simulink model "LQI_tests"  (R2026a)
settings: Solver=FixedStepAuto  StopTime=60  FixedStep=1e-3  RelTol=1e-5
values from neighbouring files (symbols this model uses):
  g = p.g    [HopperLinearization_6DOF.m]    (also in HopperLinearization_6DOF_LQR.m; HopperLinearization_6DOF_inertial.m; HopperLinearization_errorq.m; TetherTrajectory.m = 9.81)
  m = p.m    [HopperLinearization_6DOF.m]    (also in HopperLinearization_6DOF_LQR.m = 114; HopperLinearization_6DOF_inertial.m = mass; HopperLinearization_errorq.m = mass; TetherTrajectory.m = m0 + (mf-m0)*(t/t_end))
  p = Simulink.Parameter(v); p.DataType = 'double'; p.StorageClass = 'Auto'    [compare_sims.m]
undefined symbols (not defined in the file or in its folder): IN, KlqI, VEH
libraries: simulink_extras x3, SignalEditorBlockLib x2, matrix_library x2, aerolibanim x1
settings Model: Creator=asing  LastModifiedBy=maxma
settings DebuggingCC: SignalInfNanChecking=warning
settings SimscapeCC: SimscapeNominalValues="[{\"value\":\"1\",\"unit\":\"A\"},{\"value\":\"1\",\"unit\":\"bar\"},{\"value\":\"1\",\"unit\":\"cm^2\"},{\"value\":\"1\",\"unit\":\"cm^3/s\"},{\"value\":\"1\",\"unit\":\"kJ/kg\"},{\"value\":\"1\",\"unit\":\"kW\"},{\"value\":\"1\",\"unit\":\"l\"},{\"value\":\"1\",\"unit\":\"N\"},{\"value\":\"1\",\"unit\":\"N*m\"},{\"value\":\"1\",\"unit\":\"V\"}]"  SimscapeLogType=none  SimscapeLogDataHistory=5000.0

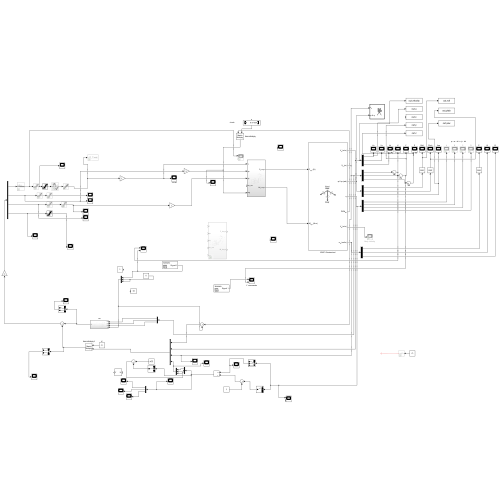
[thumbnail: Simulink's stored preview of the top-level diagram]
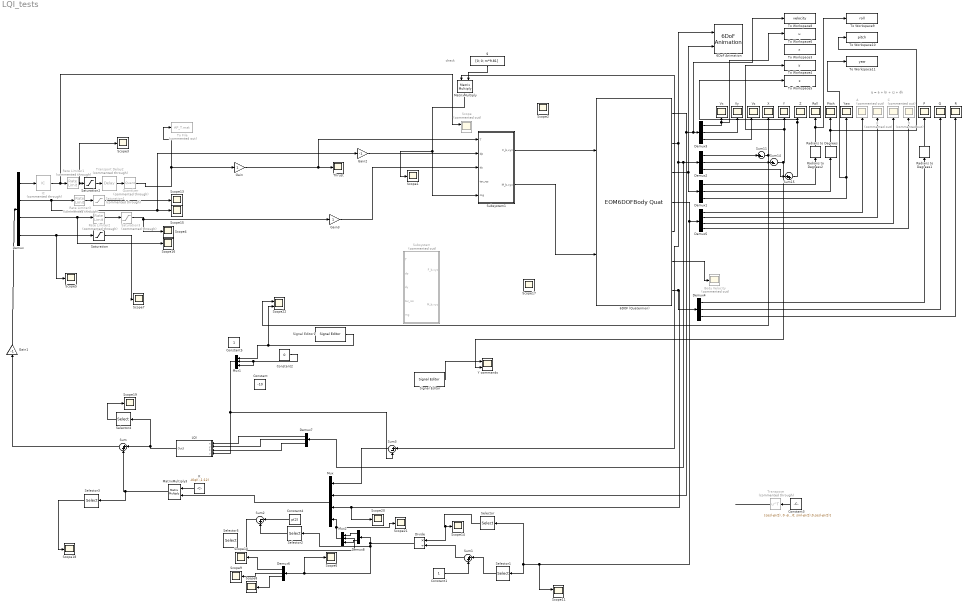
== system LQI_tests ==
  note: check
  note: q = a + bi + cj + dk
  6DOF (Quaternion) : EOM6DOFBodyQuat  eul_0=[0 pi/2 0]  inertia=[1 0 0; 0 4 0; 0 0 4]
  6DoF Animation : aerolibanim/6DoF Animation  u1=[0 200 -200 200 -100 5]  u2=0.1  u3=2  u4=[4000 0 -5000]  u5=Fixed position  u6=[100 100 -50]  u7=10  u8=on
  A : Scope  Commented=on
      settings: ActiveDisplayYMinimum=-1  ActiveDisplayYMaximum=1  DataLoggingVariableName=ScopeData12
  B : Scope  Commented=on
      settings: ActiveDisplayYMinimum=-1  ActiveDisplayYMaximum=1  DataLoggingVariableName=ScopeData13
  Body Velocity : Scope  Commented=on
      settings: ActiveDisplayYMinimum=-9.910378836747423  ActiveDisplayYMaximum=88.214312640198585  DataLoggingVariableName=ScopeData29
  C : Scope  Commented=on
      settings: DataLoggingVariableName=ScopeData14
  Constant : Constant  Value=-10
  Constant1 : Constant
  Constant2 : Constant  Value=0
  Constant3 : Constant  Value=[cos(-pi/2), 0 -sin(-pi/2); 0, 1, 0; sin(-pi/2),0,cos(-pi/2)]
  Constant4 : Constant  Value=p(2)
  Constant5 : Constant
  D : Scope  Commented=on
      settings: DataLoggingVariableName=ScopeData15
  Demux : Demux
  Demux{1..4,6..8} (7 alike) : Demux  Outputs=3
  Demux5 : Demux
  Divide : Product  Inputs=*/
  Gain : Gain
  Gain1 : Gain  Gain=-1
  Gain2 : Gain  Gain=-1
  Gain3 : Gain
  IC : InitialCondition  Commented=through  Value=VEH.mass.wet*g
  K : Constant  Value=-KlqI(:,1:12)
  LQI : Subsystem
  MatrixMultiply : Product  Multiplication=Matrix(*)
  MatrixMultiply3 : Product  Multiplication=Matrix(*)
  Mux : Mux
  Mux1 : Mux  Inputs=3
  Mux2 : Mux  Inputs=3
  P : Scope
      settings: ActiveDisplayYMinimum=-8.26326566221206E-12  ActiveDisplayYMaximum=2.9451140456166085E-11  DataLoggingVariableName=ScopeData9
  Pitch : Scope
      settings: ActiveDisplayYMinimum=87.618751786156409  ActiveDisplayYMaximum=90.264583134871515  DataLoggingVariableName=ScopeData4
  Q : Scope
      settings: ActiveDisplayYMinimum=-1  ActiveDisplayYMaximum=1  DataLoggingVariableName=ScopeData10
  Quantizer : Quantizer  Commented=through  QuantizationInterval=IN.throttle_valve.resolution
  R : Scope
      settings: ActiveDisplayYMinimum=-0.0070860969112896514  ActiveDisplayYMaximum=0.0085398632976064828  DataLoggingVariableName=ScopeData11
  Radians to Degrees : simulink_extras/Transformations/Radians to Degrees
  Radians to Degrees1 : simulink_extras/Transformations/Radians to Degrees
  Radians to Degrees2 : simulink_extras/Transformations/Radians to Degrees
  Rate Limiter1 : RateLimiter  Commented=through  RisingSlewLimit=10  FallingSlewLimit=-10  SampleTimeMode=inherited
  Rate Limiter2 : RateLimiter  Commented=through  RisingSlewLimit=pi/16  FallingSlewLimit=-pi/16  SampleTimeMode=inherited
  Rate Limiter3 : RateLimiter  Commented=through  RisingSlewLimit=pi/16  FallingSlewLimit=-pi/16  SampleTimeMode=inherited
  Roll : Scope
      settings: ActiveDisplayYMinimum=-224.12991219773974  ActiveDisplayYMaximum=188.93119763422254  DataLoggingVariableName=ScopeData3
  Saturation : Saturate  UpperLimit=50  LowerLimit=-50
  Saturation1 : Saturate  Commented=through  UpperLimit=pi/16  LowerLimit=-pi/16
  Saturation2 : Saturate  UpperLimit=20  LowerLimit=-20
  Saturation3 : Saturate  Commented=through  UpperLimit=pi/16  LowerLimit=-pi/16
  Scope : Scope  Commented=on  NumInputPorts=2
      settings: ActiveDisplayYMinimum=725.64918679567745  ActiveDisplayYMaximum=1423.3753088923004  DataLoggingVariableName=ScopeData52
  Scope{1..10,13..21} (19 alike) : Scope
      Scope1 settings: ActiveDisplayYMinimum=-1  ActiveDisplayYMaximum=1  DataLoggingVariableName=ScopeData31
      Scope10 settings: ActiveDisplayYMinimum=-4.9890047199405645  ActiveDisplayYMaximum=5.2625297562526274  DataLoggingVariableName=ScopeData24
      Scope13 settings: ActiveDisplayYMinimum=-0.011880947650151304  ActiveDisplayYMaximum=0.017843667196405844  DataLoggingVariableName=ScopeData32
      Scope14 settings: ActiveDisplayYMinimum=-1  ActiveDisplayYMaximum=1  DataLoggingVariableName=ScopeData30
      Scope15 settings: ActiveDisplayYMinimum=-0.011880947650151304  ActiveDisplayYMaximum=0.017843667196405844  DataLoggingVariableName=ScopeData33
      Scope16 settings: ActiveDisplayYMinimum=-2.0834911405645039E-9  ActiveDisplayYMaximum=2.3149901561827815E-10  DataLoggingVariableName=ScopeData34
      Scope17 settings: ActiveDisplayYMinimum=-1  ActiveDisplayYMaximum=1  DataLoggingVariableName=ScopeData35
      Scope18 settings: ActiveDisplayYMinimum=-0.0038539564118753185  ActiveDisplayYMaximum=0.0039515634067714732  DataLoggingVariableName=ScopeData38
      Scope19 settings: ActiveDisplayYMinimum=-1  ActiveDisplayYMaximum=1  DataLoggingVariableName=ScopeData39
      Scope2 settings: ActiveDisplayYMinimum=-2.15049803632378E+91  ActiveDisplayYMaximum=8.000199525245886E+91  DataLoggingVariableName=ScopeData16
      Scope20 settings: ActiveDisplayYMinimum=-0.014597073503933574  ActiveDisplayYMaximum=0.011710976990840343  DataLoggingVariableName=ScopeData36
      Scope21 settings: ActiveDisplayYMinimum=-1  ActiveDisplayYMaximum=1  DataLoggingVariableName=ScopeData37
      Scope3 settings: ActiveDisplayYMinimum=-14.409381539432603  ActiveDisplayYMaximum=1.6010423932702889  DataLoggingVariableName=ScopeData17
      Scope4 settings: ActiveDisplayYMinimum=-0.22093678843770853  ActiveDisplayYMaximum=0.0249356874457561  DataLoggingVariableName=ScopeData18
      Scope5 settings: ActiveDisplayYMinimum=-59.073001162491146  ActiveDisplayYMaximum=98.278860989440048  DataLoggingVariableName=ScopeData27
      Scope6 settings: ActiveDisplayYMinimum=-0.051776695296636865  ActiveDisplayYMaximum=0.4659902576697319  DataLoggingVariableName=ScopeData21
      Scope7 settings: ActiveDisplayYMinimum=-62.5  ActiveDisplayYMaximum=62.5  DataLoggingVariableName=ScopeData62
      Scope8 settings: ActiveDisplayYMinimum=-2.1309134727823871  ActiveDisplayYMaximum=1.9654214801927952  DataLoggingVariableName=ScopeData22
      Scope9 settings: ActiveDisplayYMinimum=-2187.3368047164704  ActiveDisplayYMaximum=295.01020706287159  DataLoggingVariableName=ScopeData23
  Scope11 : Scope  NumInputPorts=2
      settings: ActiveDisplayYMinimum=-1.2499999748076374  ActiveDisplayYMaximum=1.2499999972008486  DataLoggingVariableName=ScopeData26
  Scope22 : Scope  NumInputPorts=2
      settings: ActiveDisplayYMinimum=-36.734345515294429  ActiveDisplayYMaximum=20.819130872097  DataLoggingVariableName=ScopeData40
  Selector : Selector  InputPortWidth=4  IndexOptions=Index vector (dialog)  Indices=[2 3 4]  OutputSizes=1
  Selector1 : Selector  InputPortWidth=4  IndexOptions=Index vector (dialog)  Indices=[1]  OutputSizes=1
  Selector2 : Selector  InputPortWidth=3  IndexOptions=Index vector (dialog)  Indices=[2]  OutputSizes=1
  Selector3 : Selector  InputPortWidth=4  IndexOptions=Index vector (dialog)  Indices=[2 3]  OutputSizes=1
  Selector4 : Selector  InputPortWidth=4  IndexOptions=Index vector (dialog)  Indices=[2 3]  OutputSizes=1
  Selector5 : Selector  NumberOfDimensions=2  InputPortWidth=3  IndexOptions=Index vector (dialog),Index vector (dialog)  Indices=[1 3],1  OutputSizes=1,1
  Signal Editor : SignalEditorBlockLib/Signal Editor  FileName=C:\Users\maxma\OneDrive\Desktop\gittest\hopper\sims\Controls Dev Test\lqitestSteps.mat  ActiveScenario=Scenario  ActiveSignal=Signal 1  IsBus=off  OutputBusObjectStr=Bus: BusObject  SampleTime=0  ZeroCross=off  OutputAfterFinalValue=Setting to zero  Unit=inherit  PreserveSignalName=on  ApplySigPropsToAllScenarios=on  ApplySigPropsToAllSignals=off  SignalPropertySource=Dialog parameters
  Signal Editor1 : SignalEditorBlockLib/Signal Editor  FileName=C:\Users\maxma\OneDrive\Desktop\gittest\hopper\sims\Controls Dev Test\lqitestSteps.mat  ActiveScenario=Scenario  ActiveSignal=Signal 1  IsBus=off  OutputBusObjectStr=Bus: BusObject  SampleTime=0  ZeroCross=off  OutputAfterFinalValue=Setting to zero  Unit=inherit  PreserveSignalName=on  ApplySigPropsToAllScenarios=on  ApplySigPropsToAllSignals=off  SignalPropertySource=Dialog parameters
  Subsystem : Subsystem  Commented=on
  Subsystem1 : Subsystem
  Sum : Sum  Inputs=|++
  Sum1 : Sum  Inputs=|++
  Sum11 : Sum  Inputs=|+-
  Sum14 : Sum  Inputs=|+-
  Sum15 : Sum  Inputs=|++
  Sum2 : Sum  Inputs=|-+
  Sum3 : Sum  Inputs=|+-
  Thrust : Scope
      settings: ActiveDisplayYMinimum=0.53330784427989109  ActiveDisplayYMaximum=13.594880195297881  DataLoggingVariableName=ScopeData25
  To File : ToFile  Commented=on  Filename=AP_T.mat  SaveFormat=Timeseries
  To Workspace10 : ToWorkspace  VariableName=pitch  SaveFormat=Timeseries  SampleTime=-1
  To Workspace11 : ToWorkspace  VariableName=yaw  SaveFormat=Timeseries  SampleTime=-1
  To Workspace3 : ToWorkspace  VariableName=x  SaveFormat=Timeseries  SampleTime=-1
  To Workspace4 : ToWorkspace  VariableName=y  SaveFormat=Timeseries  SampleTime=-1
  To Workspace5 : ToWorkspace  VariableName=z  SaveFormat=Timeseries  SampleTime=-1
  To Workspace6 : ToWorkspace  VariableName=u  SaveFormat=Timeseries  SampleTime=-1
  To Workspace8 : ToWorkspace  VariableName=velocity  SaveFormat=Timeseries  SampleTime=-1
  To Workspace9 : ToWorkspace  VariableName=roll  SaveFormat=Timeseries  SampleTime=-1
  Transport Delay2 : TransportDelay  Commented=through  DelayTime=IN.throttle_valve_latency
  Transpose : Math  Commented=through  Operator=transpose
  Vx : Scope
      settings: ActiveDisplayYMinimum=-63.872379284445891  ActiveDisplayYMaximum=574.47074934538614  DataLoggingVariableName=ScopeData6
  Vy : Scope
      settings: ActiveDisplayYMinimum=-1  ActiveDisplayYMaximum=1  DataLoggingVariableName=ScopeData7
  Vz : Scope  NumInputPorts=2
      settings: ActiveDisplayYMinimum=-39.057978029142859  ActiveDisplayYMaximum=300.25377175337246  DataLoggingVariableName=ScopeData8
  X : Scope
      settings: ActiveDisplayYMinimum=-2.0444125415499856  ActiveDisplayYMaximum=1.2987978569688314
  Y : Scope
      settings: ActiveDisplayYMinimum=-0.93800150729530174  ActiveDisplayYMaximum=8.4409024914672273
  Y commands : Scope  NumInputPorts=2
      settings: ActiveDisplayYMinimum=-1.125  ActiveDisplayYMaximum=0.12499999999999997  DataLoggingVariableName=ScopeData19
  Yaw : Scope
      settings: ActiveDisplayYMinimum=-2.1621937540646594  ActiveDisplayYMaximum=1.7043365978662512  DataLoggingVariableName=ScopeData5
  Z : Scope  NumInputPorts=2
      settings: ActiveDisplayYMinimum=-0.57646211856596  ActiveDisplayYMaximum=2.6247212976912433  DataLoggingVariableName=ScopeData2
  g : Constant  Value=[0; 0; m*9.81]
  wires:
  6DOF (Quaternion)/3 -> Demux1/1, 6DoF Animation/2
  Demux1/2 -> Radians to Degrees/1
  Demux3/1 -> To Workspace6/1, Vx/1
  Demux3/2 -> Vy/1
  6DOF (Quaternion)/4 -> Scope11/1, Selector/1, Selector1/1, Demux5/1
  Demux4/1 -> Radians to Degrees1/1
  Demux4/2 -> Q/1
  Demux4/3 -> R/1
  Demux5/1 -> A/1
  Demux5/2 -> B/1
  Demux5/3 -> C/1
  Demux5/4 -> D/1
  Demux3/3 -> Vz/1
  6DOF (Quaternion)/6 -> Body Velocity/1
  Demux1/1 -> Radians to Degrees2/1
  Demux1/3 -> Yaw/1, To Workspace11/1
  g/1 -> MatrixMultiply/2
  Rate Limiter1/1 -> Scope3/1, Saturation2/1
  Demux/2 -> Rate Limiter3/1, Gain2/1, Scope15/1
  Demux/1 -> IC/1
  Transport Delay2/1 -> Quantizer/1
  IC/1 -> Scope/1, Rate Limiter1/1
  6DOF (Quaternion)/1 -> Mux/2, To Workspace8/1, Demux3/1
  6DOF (Quaternion)/2 -> Sum3/1, Demux7/1, Demux2/1, 6DoF Animation/1
  Saturation2/1 -> Transport Delay2/1
  Demux2/1 -> Sum11/1
  Demux2/2 -> Sum14/1
  Sum14/1 -> Y commands/2, To Workspace4/1, Y/1
  Demux2/3 -> Sum15/1
  Demux/4 -> Scope5/1, Saturation/1
  Radians to Degrees/1 -> To Workspace10/1, Pitch/1
  Sum15/1 -> To Workspace5/1, Z/1
  Radians to Degrees1/1 -> P/1
  Radians to Degrees2/1 -> To Workspace9/1, Roll/1
  6DOF (Quaternion)/5 -> MatrixMultiply/1
  Demux7/3 -> LQI/3(z)
  Mux/1 -> MatrixMultiply3/2
  MatrixMultiply3/1 -> Selector3/1, Sum/2
  K/1 -> MatrixMultiply3/1
  Quantizer/1 -> To File/1, Gain/1
  Signal Editor/1 -> Y commands/1
  Sum/1 -> Gain1/1
  Gain/1 -> Subsystem1/1(T), Thrust/1
  Demux/3 -> Scope16/1, Rate Limiter2/1
  Gain1/1 -> Demux/1
  Demux7/2 -> LQI/2(y)
  Demux7/1 -> LQI/1(x)
  Mux1/1 -> LQI/4(r), Sum3/2
  LQI/1(Out3) -> Selector4/1, Sum/1
  Sum11/1 -> X/1, Scope22/1
  Demux6/3 -> Scope8/1
  Demux6/2 -> Scope9/1
  Demux6/1 -> Scope10/1
  Selector/1 -> Divide/1, Scope14/1
  Constant1/1 -> Sum1/2
  Selector1/1 -> Sum1/1
  Sum1/1 -> Divide/2
  Divide/1 -> Scope6/1, Demux6/1, Selector2/1, Demux8/1
  Constant3/1 -> Transpose/1
  Transpose/1 -> ?
  MatrixMultiply/1 -> Subsystem1/5(mg), Scope1/1
  Selector3/1 -> Scope18/1
  Selector4/1 -> Scope19/1
  Selector2/1 -> Sum2/2
  Demux8/3 -> Mux2/3
  Demux8/1 -> Mux2/1
  Sum3/1 -> Mux/1
  Saturation/1 -> Scope7/1
  Saturation3/1 -> Scope4/1, Gain3/1
  6DOF (Quaternion)/7 -> Demux4/1, Scope20/1, Mux/3
  Saturation1/1 -> Scope13/1
  Rate Limiter3/1 -> Saturation1/1
  Rate Limiter2/1 -> Saturation3/1
  Constant2/1 -> Mux1/2, Mux1/3
  Constant4/1 -> Sum2/1
  Subsystem1/1(F_b,xyz) -> 6DOF (Quaternion)/1
  Subsystem1/2(M_b,xyz) -> 6DOF (Quaternion)/2
  Mux2/1 -> Mux/4, Scope21/1
  Sum2/1 -> Mux2/2
  Signal Editor1/1 -> Scope22/2, Mux1/1
  Gain2/1 -> Subsystem1/2(dp)
  Gain3/1 -> Subsystem1/3(dy)

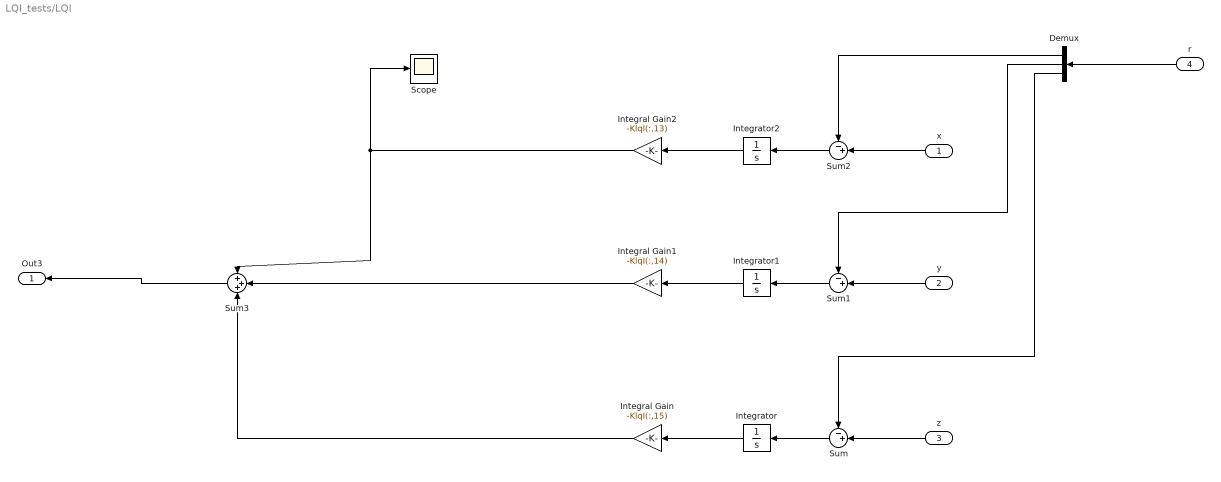
== system LQI_tests/LQI ==
  x : Inport
  y : Inport  Port=2
  z : Inport  Port=3
  r : Inport  Port=4
  Demux : Demux  Outputs=3
  Integral Gain : Gain  Gain=-KlqI(:,15)
  Integral Gain1 : Gain  Gain=-KlqI(:,14)
  Integral Gain2 : Gain  Gain=-KlqI(:,13)
  Integrator : Integrator
  Integrator1 : Integrator
  Integrator2 : Integrator
  Scope : Scope
      settings: ActiveDisplayYMinimum=-1  ActiveDisplayYMaximum=1  DataLoggingVariableName=ScopeData20
  Sum : Sum  Inputs=-+|
  Sum1 : Sum  Inputs=-+|
  Sum2 : Sum  Inputs=-+|
  Sum3 : Sum  Inputs=+++
  Out3 : Outport
  wires:
  z/1 -> Sum/2
  Sum/1 -> Integrator/1
  Integrator/1 -> Integral Gain/1
  Integral Gain/1 -> Sum3/3
  Integral Gain1/1 -> Sum3/2
  Integrator1/1 -> Integral Gain1/1
  Sum1/1 -> Integrator1/1
  y/1 -> Sum1/2
  Integral Gain2/1 -> Sum3/1, Scope/1
  Integrator2/1 -> Integral Gain2/1
  Sum2/1 -> Integrator2/1
  x/1 -> Sum2/2
  r/1 -> Demux/1
  Demux/1 -> Sum2/1
  Demux/2 -> Sum1/1
  Demux/3 -> Sum/1
  Sum3/1 -> Out3/1

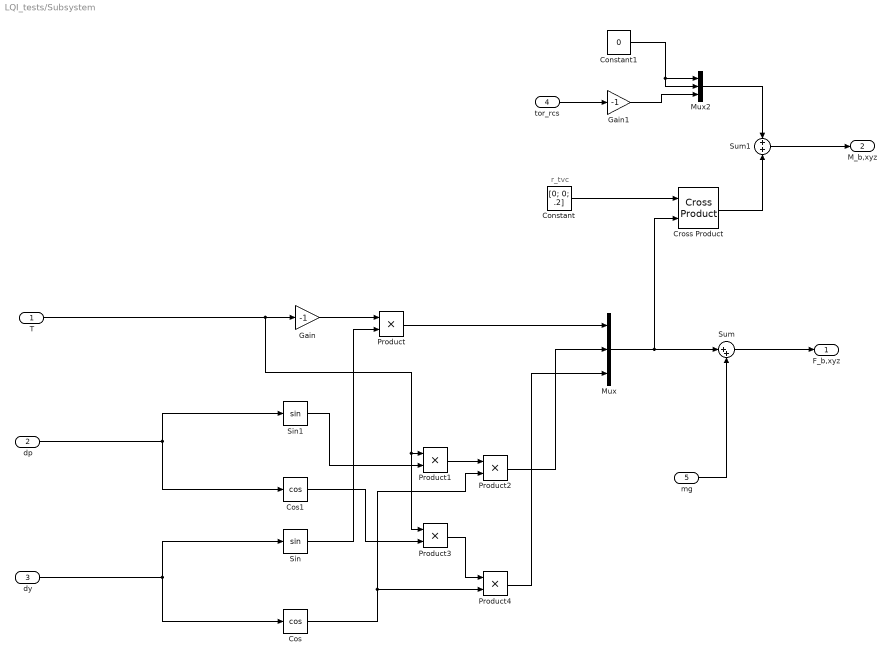
== system LQI_tests/Subsystem ==
  note: r_tvc
  T : Inport
  dp : Inport  Port=2
  dy : Inport  Port=3
  tor_rcs : Inport  Port=4
  mg : Inport  Port=5
  Constant : Constant  Value=[0; 0; .2]
  Constant1 : Constant  Value=0
  Cos : Trigonometry  Operator=cos
  Cos1 : Trigonometry  Operator=cos
  Cross Product : matrix_library/Cross Product
  Gain : Gain  Gain=-1
  Gain1 : Gain  Gain=-1
  Mux : Mux  Inputs=3
  Mux2 : Mux  Inputs=3
  Product{,1..4} (5 alike) : Product
  Sin : Trigonometry
  Sin1 : Trigonometry
  Sum : Sum  Inputs=|++
  Sum1 : Sum  Inputs=+|+
  F_b,xyz : Outport
  M_b,xyz : Outport  Port=2
  wires:
  T/1 -> Product3/1, Product1/1, Gain/1
  dy/1 -> Cos/1, Sin/1
  Gain/1 -> Product/1
  Sin/1 -> Product/2
  Product/1 -> Mux/1
  dp/1 -> Cos1/1, Sin1/1
  Sin1/1 -> Product1/2
  Cos/1 -> Product4/2, Product2/2
  Product1/1 -> Product2/1
  Cos1/1 -> Product3/2
  Product3/1 -> Product4/1
  Product4/1 -> Mux/3
  Product2/1 -> Mux/2
  Mux/1 -> Sum/1, Cross Product/2
  Constant/1 -> Cross Product/1
  mg/1 -> Sum/2
  Constant1/1 -> Mux2/2, Mux2/1
  Gain1/1 -> Mux2/3
  tor_rcs/1 -> Gain1/1
  Mux2/1 -> Sum1/1
  Cross Product/1 -> Sum1/2
  Sum/1 -> F_b,xyz/1
  Sum1/1 -> M_b,xyz/1

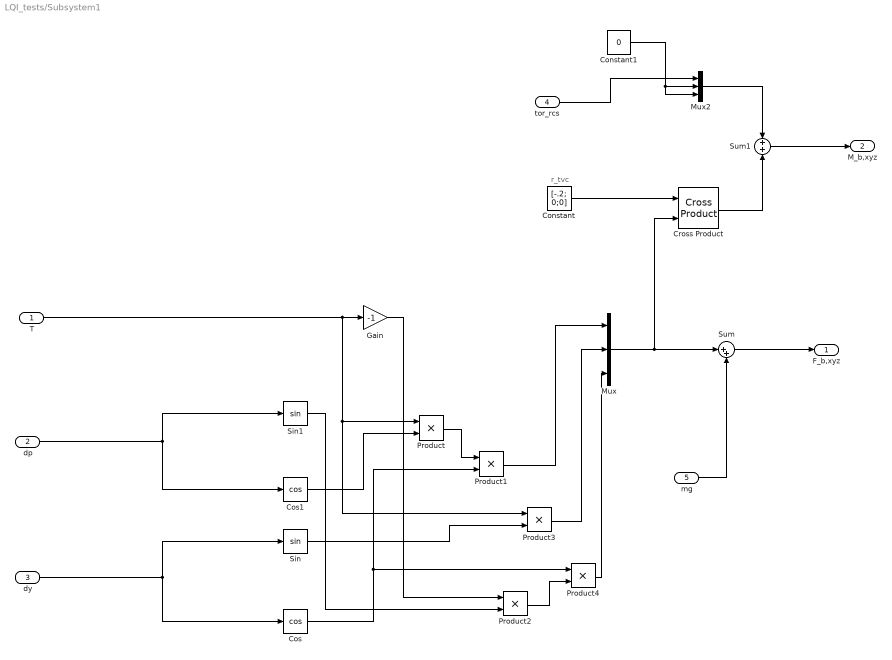
== system LQI_tests/Subsystem1 ==
  note: r_tvc
  T : Inport
  dp : Inport  Port=2
  dy : Inport  Port=3
  tor_rcs : Inport  Port=4
  mg : Inport  Port=5
  Constant : Constant  Value=[-.2; 0;0]
  Constant1 : Constant  Value=0
  Cos : Trigonometry  Operator=cos
  Cos1 : Trigonometry  Operator=cos
  Cross Product : matrix_library/Cross Product
  Gain : Gain  Gain=-1
  Mux : Mux  Inputs=3
  Mux2 : Mux  Inputs=3
  Product{,1..4} (5 alike) : Product
  Sin : Trigonometry
  Sin1 : Trigonometry
  Sum : Sum  Inputs=|++
  Sum1 : Sum  Inputs=+|+
  F_b,xyz : Outport
  M_b,xyz : Outport  Port=2
  wires:
  T/1 -> Product3/1, Product/1, Gain/1
  dy/1 -> Cos/1, Sin/1
  dp/1 -> Cos1/1, Sin1/1
  Mux/1 -> Sum/1, Cross Product/2
  Constant/1 -> Cross Product/1
  mg/1 -> Sum/2
  Constant1/1 -> Mux2/3, Mux2/2
  tor_rcs/1 -> Mux2/1
  Mux2/1 -> Sum1/1
  Cross Product/1 -> Sum1/2
  Sum/1 -> F_b,xyz/1
  Sum1/1 -> M_b,xyz/1
  Cos1/1 -> Product/2
  Cos/1 -> Product4/1, Product1/2
  Product/1 -> Product1/1
  Product1/1 -> Mux/1
  Sin/1 -> Product3/2
  Product3/1 -> Mux/2
  Gain/1 -> Product2/1
  Sin1/1 -> Product2/2
  Product2/1 -> Product4/2
  Product4/1 -> Mux/3
